simulink library "Valve_table"  (R2018b)
settings: Solver=ode45  StartTime=0.0  StopTime=10.0  RelTol=1e-3  EnableMultiTasking=on
undefined symbols (not defined in the file): DPConstant, DPLinear, DPQuadratic, ID, Pressure
libraries: carnot x2
settings Model: Creator=lena.frank  LastModifiedBy=P41573
settings DataIOCC: LimitDataPoints=on  SaveFormat=Array  SignalLoggingSaveFormat=ModelDataLogs
settings OptimizationCC: ExpressionDepthLimit=2147483647  LifeSpan=inf
settings DebuggingCC: UnderspecifiedInitializationDetection=Classic  MergeDetectMultiDrivingBlocksExec=none  SolverPrmCheckMsg=warning  FcnCallInpInsideContextMsg=warning  StateNameClashWarn=warning  SFUnexpectedBacktrackingDiag=warning  SFNoUnconditionalDefaultTransitionDiag=warning  SFExecutionAtInitializationDiag=none
settings HardwareCC: ProdBitPerPointer=32  ProdBitPerSizeT=32  ProdBitPerPtrDiffT=32  ProdLargestAtomicFloat=None  ProdIntDivRoundTo=Undefined  ProdEndianess=Unspecified  ProdWordSize=32  ProdHWDeviceType=32-bit Generic
settings ModelReferenceCC: PropagateSignalLabelsOutOfModel=off
settings SFSimCC: SimUseLocalCustomCode=off
settings RTWCC: RTWUseLocalCustomCode=off
settings CodeAppCC: StateflowObjectComments=on
settings GRTTargetCC: TargetLangStandard=C89/C90 (ANSI)  GeneratePreprocessorConditionals=Disable all  CombineOutputUpdateFcns=off  GRTInterface=on
settings ConfigComp: CovMetricSettings=dw  CovHtmlReporting=on  CovSaveCumulativeToWorkspaceVar=on  CovSaveSingleToWorkspaceVar=on  CovExternalEMLEnable=off

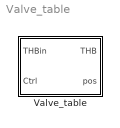
== system Valve_table ==
  Valve_table : Subsystem  mask(Valve Function){h=[0 1], psi=[0.04 1], kvs=0.9, dt_V=0.01}
      mask prompts: h "Ctrl: relative valve position data (vector)"; psi "Psi: relative flow coefficient data - vector of length(Ctrl)"; kvs "Kvs: flow coefficient of the open valve in m³/h"; dt_V "Valve running time in s"
      mask help:
      | Model of a valve with a lookup table for the flow coefficient characteristic:
      |   psi = lookuptable(h)
      | with
      |   h = H/H100   relative opening
      |   Kv                 flow coefficient in m³/h
      |   Kv = Vdot * sqrt(1e5Pa/dp * density/1000kg/m³)
      |   Kvs                flow coefficient  in m³/h of the fully opened valve.
      |   psi = Kv/Kvs  relative flow coefficient
      |   Vdot             volumetric flow rate in m³/h
      | Note: Psi must be > 0 for Ctrl = 0
      | Typical value for the relative flow coefficient at zero opening psi_0 is 0.04
      mask Help: web(fullfile(path_carnot('help'),'Valve_table.html'),'-helpbrowser')
      mask TypeOptions h: h2psi_table/BreakpointsForDimension1
      mask TypeOptions psi: h2psi_table/Table
      mask TypeOptions kvs: relFlowCoeff2qua/kvs
      mask TypeOptions dt_V: Rate Limiter/dt_V
      mask Display:
      | plot(-30,-20,130,120,[10,90,90,10,10],[50,0,50,0,50],...
      |     [50,50],[50,25],...
      |     [40,30,30,40,60,70,70,60,40],[50,60,80,90,90,80,60,50,50],...
      |     [60,60,50,40,40],[60,80,70,80,60])

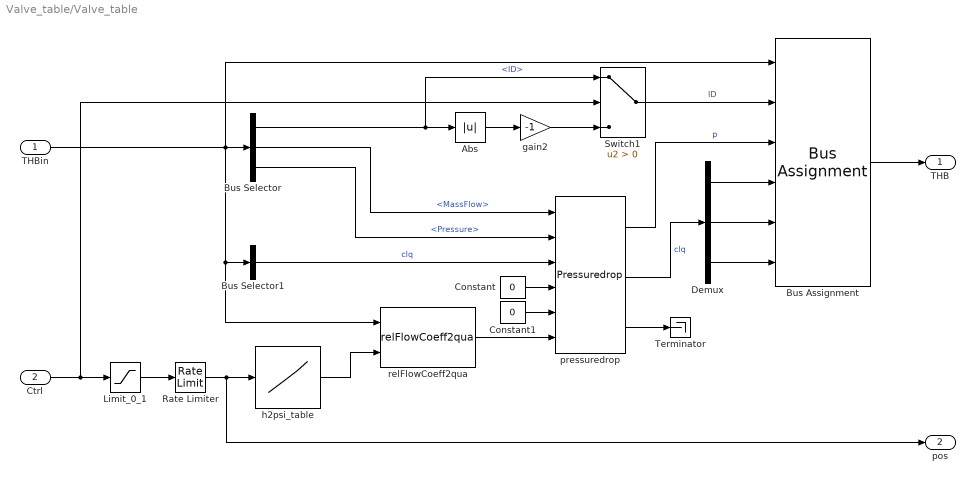
== system Valve_table/Valve_table ==
  THBin : Inport
  Ctrl : Inport  Port=2
  Abs : Abs
  Bus Assignment : BusAssignment  AssignedSignals=ID,Pressure,DPConstant,DPLinear,DPQuadratic
  Bus Selector : BusSelector  OutputSignals=ID,MassFlow,Pressure
  Bus Selector1 : BusSelector  OutputSignals=DPConstant,DPLinear,DPQuadratic  OutputAsBus=on
  Constant : Constant  Value=0
  Constant1 : Constant  Value=0
  Demux : Demux  Outputs=3
  Limit_0_1 : Saturate  UpperLimit=1  LowerLimit=0
  Rate Limiter : RateLimiter  RisingSlewLimit=1/dt_V  FallingSlewLimit=-1/dt_V  SampleTimeMode=inherited  mask{dt_V=dt_V}
      mask prompts: dt_V "Valve running time in s"
  Switch1 : Switch  Criteria=u2 > Threshold  SaturateOnIntegerOverflow=on  InputSameDT=on
  Terminator : Terminator
  gain2 : Gain  Gain=-1  SaturateOnIntegerOverflow=on  OutDataTypeStr=Inherit: Same as input  ParamDataTypeStr=Inherit: Same as input
  h2psi_table : Lookup_n-D  NumberOfTableDimensions=1  BreakpointsForDimension1=h  Table=psi  InternalRulePriority=Speed  RndMeth=Simplest  InputSameDT=on
  pressuredrop : carnot/Basic/Pressure_Drop/Pressuredrop
      settings: SourceProductName=Carnot
  relFlowCoeff2qua : carnot/Basic/Pressure_Drop/relFlowCoeff2qua  kvs=kvs
      settings: SourceProductName=Carnot
  THB : Outport
  pos : Outport  Port=2
  wires:
  Rate Limiter/1 -> pos/1, h2psi_table/1
  relFlowCoeff2qua/1 -> pressuredrop/6
  Limit_0_1/1 -> Rate Limiter/1
  h2psi_table/1 -> relFlowCoeff2qua/2
  gain2/1 -> Switch1/3
  Bus Selector/1 -> Switch1/1, Abs/1  "<ID>"
  Ctrl/1 -> Limit_0_1/1, Switch1/2
  Bus Selector1/1 -> pressuredrop/3  "clq"
  pressuredrop/1 -> Bus Assignment/3  "p"
  Bus Selector/2 -> pressuredrop/1  "<MassFlow>"
  Switch1/1 -> Bus Assignment/2  "ID"
  Abs/1 -> gain2/1
  Bus Selector/3 -> pressuredrop/2  "<Pressure>"
  pressuredrop/2 -> Demux/1  "clq"
  Constant/1 -> pressuredrop/4
  Constant1/1 -> pressuredrop/5
  pressuredrop/3 -> Terminator/1
  THBin/1 -> Bus Selector/1, relFlowCoeff2qua/1, Bus Selector1/1, Bus Assignment/1
  Bus Assignment/1 -> THB/1
  Demux/1 -> Bus Assignment/4
  Demux/2 -> Bus Assignment/5
  Demux/3 -> Bus Assignment/6
